simulink model "escontrol"  (R2024a)
settings: configuration reference "Configuration_template" (kept outside this file)
undefined symbols (not defined in the file): a, b, enable_hpf, enable_lpf, k, phi1, phi2, theta0, theta_max, theta_min, w, w_hpf, w_lpf
libraries: escontroller_lib x2
settings Model: DataDictionary=escontrol.sldd  Creator=tkigezi  LastModifiedBy=tn212
settings ConfigSetRef: SourceName=Configuration_template

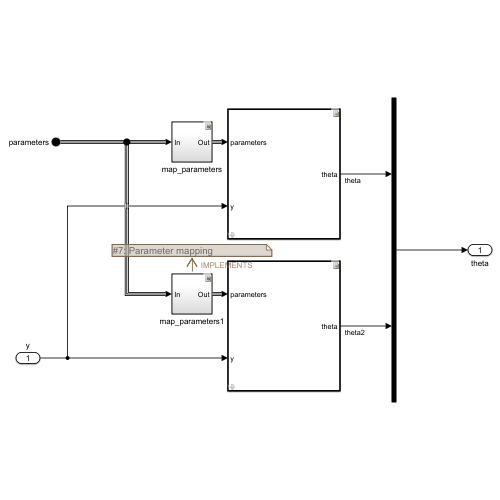
[thumbnail: Simulink's stored preview of the top-level diagram]
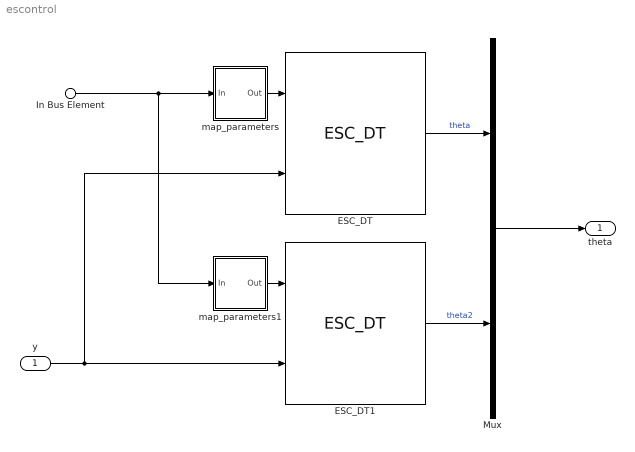
== system escontrol ==
  y : Inport
  In Bus Element : Inport  Port=2  PortName=parameters
  ESC_DT : escontroller_lib/ESC_DT  offset_sinwave_modulation=0  offset_sinwave_demodulation=0
  ESC_DT1 : escontroller_lib/ESC_DT  offset_sinwave_modulation=0  offset_sinwave_demodulation=0
  Mux : Mux  Inputs=2
  map_parameters : Subsystem
  map_parameters1 : Subsystem
  theta : Outport
  wires:
  ESC_DT1/1 -> Mux/2  "theta2"
  Mux/1 -> theta/1
  ESC_DT/1 -> Mux/1  "theta"
  In Bus Element/1 -> map_parameters1/1(In), map_parameters/1(In)
  map_parameters1/1(Out) -> ESC_DT1/1
  map_parameters/1(Out) -> ESC_DT/1
  y/1 -> ESC_DT1/2, ESC_DT/2

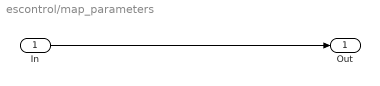
== system escontrol/map_parameters ==
  In : Inport
  Out : Outport
  wires:
  In/1 -> Out/1

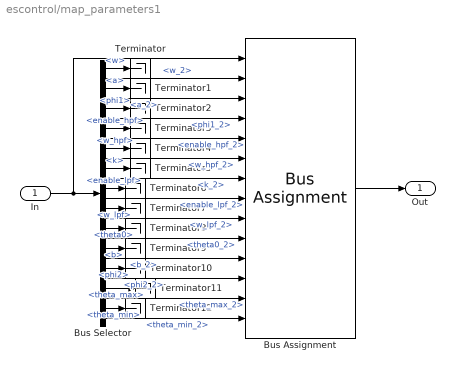
== system escontrol/map_parameters1 ==
  In : Inport
  Bus Assignment : BusAssignment  AssignedSignals=w,a,phi1,enable_hpf,w_hpf,k,enable_lpf,w_lpf,theta0,b,phi2,theta_max,theta_min
  Bus Selector : BusSelector  OutputSignals=w,w_2,a,a_2,phi1,phi1_2,enable_hpf,enable_hpf_2,w_hpf,w_hpf_2,k,k_2,enable_lpf,enable_lpf_2,w_lpf,w_lpf_2,theta0,theta0_2,b,b_2,phi2,phi2_2,theta_max,theta_max_2,theta_min,theta_min_2
  Terminator{,1..12} (13 alike) : Terminator
  Out : Outport
  wires:
  Bus Selector/15 -> Terminator7/1  "<w_lpf>"
  Bus Selector/7 -> Terminator3/1  "<enable_hpf>"
  Bus Selector/25 -> Terminator12/1  "<theta_min>"
  In/1 -> Bus Assignment/1, Bus Selector/1
  Bus Selector/11 -> Terminator5/1  "<k>"
  Bus Selector/21 -> Terminator10/1  "<phi2>"
  Bus Selector/17 -> Terminator8/1  "<theta0>"
  Bus Selector/23 -> Terminator11/1  "<theta_max>"
  Bus Selector/13 -> Terminator6/1  "<enable_lpf>"
  Bus Selector/9 -> Terminator4/1  "<w_hpf>"
  Bus Selector/1 -> Terminator/1  "<w>"
  Bus Selector/3 -> Terminator1/1  "<a>"
  Bus Selector/19 -> Terminator9/1  "<b>"
  Bus Selector/5 -> Terminator2/1  "<phi1>"
  Bus Selector/2 -> Bus Assignment/2  "<w_2>"
  Bus Selector/4 -> Bus Assignment/3  "<a_2>"
  Bus Selector/6 -> Bus Assignment/4  "<phi1_2>"
  Bus Selector/8 -> Bus Assignment/5  "<enable_hpf_2>"
  Bus Selector/10 -> Bus Assignment/6  "<w_hpf_2>"
  Bus Selector/12 -> Bus Assignment/7  "<k_2>"
  Bus Selector/14 -> Bus Assignment/8  "<enable_lpf_2>"
  Bus Selector/16 -> Bus Assignment/9  "<w_lpf_2>"
  Bus Selector/18 -> Bus Assignment/10  "<theta0_2>"
  Bus Selector/20 -> Bus Assignment/11  "<b_2>"
  Bus Selector/22 -> Bus Assignment/12  "<phi2_2>"
  Bus Selector/24 -> Bus Assignment/13  "<theta_max_2>"
  Bus Selector/26 -> Bus Assignment/14  "<theta_min_2>"
  Bus Assignment/1 -> Out/1
